simulink model "StereoImageRectificationHDL"  (R2022a)
settings: Solver=FixedStepDiscrete  StartTime=0.0  StopTime=totalPixels*totalLines  FixedStep=1  RelTol=1e-3
InitFcn:
  | load('stereoParams.mat');
  | img = imread(get_param('StereoImageRectificationHDL/LeftInputImage','FileName'));
  | dimOut=size(img);
  | [imgRowSize, imgColSize] = size(img);
  | run('ComputeRectificationParams.m');
values from neighbouring files (symbols this model uses):
  displacement = maxDev+firstRow    [ComputeRectificationParams.m]
  distCoeffsL = [this.CameraParameters1.RadialDistortion, this.CameraParameters1.TangentialDistortion]    [ComputeRectificationParams.m]
  distCoeffsR = [this.CameraParameters2.RadialDistortion, this.CameraParameters2.TangentialDistortion]    [ComputeRectificationParams.m]
  offset = displacement+50    [ComputeRectificationParams.m]
  recleftfx = 1/intrinsicL(1,1)    [ComputeRectificationParams.m]
  recleftfy = 1/intrinsicL(2,2)    [ComputeRectificationParams.m]
  recrightfx = 1/intrinsicR(1,1)    [ComputeRectificationParams.m]
  recrightfy = 1/intrinsicR(2,2)    [ComputeRectificationParams.m]
  totalLines = R + 100    (= 580)    [setup.m]
  totalPixels = C + frontPorch    (= 802)    [setup.m]
undefined symbols (not defined in the file or in its folder): gray, imgColSize, imgRowSize, intrinsicL, intrinsicR, leftH, rightH, XBounds, YBounds
libraries: simulink x62, hdlsllib x30, visionhdlio x4, visionsources x2, visionhdlutilities x1
(part 1 of 3)
settings Model: DataTypeOverride=Off  SimulationMode=accelerator  Creator=The MathWorks, Inc.  LastModifiedBy=kaputa
settings SolverCC: AlgebraicLoopSolver=TrustRegion
settings DataIOCC: SaveOutput=off  SaveTime=off
settings OptimizationCC: BlockReduction=off  ConditionallyExecuteInputs=off  DefaultParameterBehavior=Inlined
settings DebuggingCC: AlgebraicLoopMsg=error  SingleTaskRateTransMsg=error  ParameterPrecisionLossMsg=none  UnconnectedInputMsg=warning  UnconnectedOutputMsg=warning  UnconnectedLineMsg=warning  SFMachineParentedDataDiag=warning
settings HardwareCC: ProdBitPerPointer=32  ProdBitPerSizeT=32  ProdBitPerPtrDiffT=32  ProdLargestAtomicFloat=None  ProdIntDivRoundTo=Undefined  ProdEndianess=Unspecified  ProdWordSize=32  ProdHWDeviceType=ASIC/FPGA->ASIC/FPGA  TargetBitPerPointer=64  TargetBitPerSizeT=64  TargetBitPerPtrDiffT=64  TargetLongLongMode=on  TargetIntDivRoundTo=Zero  TargetEndianess=LittleEndian  TargetWordSize=64  TargetHWDeviceType=Custom Processor->MATLAB Host Computer  ProdEqTarget=off

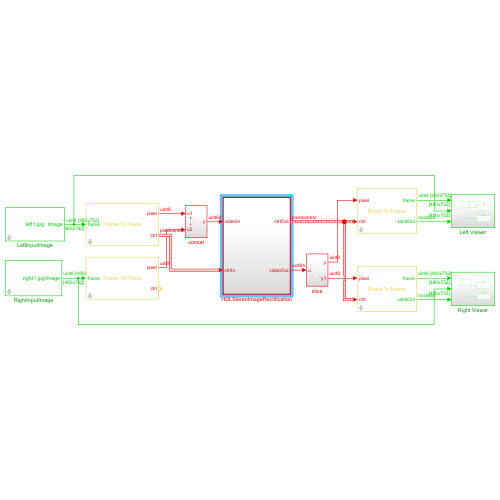
[thumbnail: Simulink's stored preview of the top-level diagram]
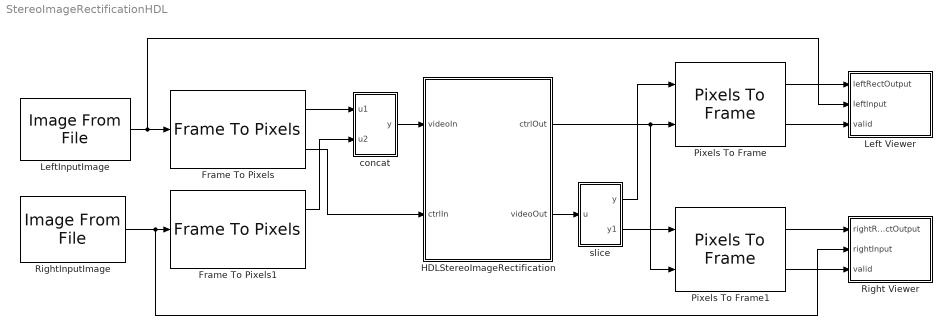
== system StereoImageRectificationHDL ==
  Frame To Pixels : visionhdlio/Frame To Pixels  NumComponents=1  NumPixels=1  VideoFormat=Custom  ActivePixelsPerLine=C  ActiveVideoLines=R  TotalPixelsPerLine=totalPixels  TotalVideoLines=totalLines  StartingActiveLine=topPorch  FrontPorch=frontPorch  SampleTime=0  VideoFormatCache=Custom  ActivePixelsPerLineCache=C  ActiveVideoLinesCache=R  TotalPixelsPerLineCache=totalPixels  TotalVideoLinesCache=totalLines  StartingActiveLineCache=topPorch  FrontPorchCache=frontPorch
      settings: SourceProductBaseCode=VT
  Frame To Pixels1 : visionhdlio/Frame To Pixels  NumComponents=1  NumPixels=1  VideoFormat=Custom  ActivePixelsPerLine=C  ActiveVideoLines=R  TotalPixelsPerLine=totalPixels  TotalVideoLines=totalLines  StartingActiveLine=topPorch  FrontPorch=frontPorch  SampleTime=0  VideoFormatCache=Custom  ActivePixelsPerLineCache=C  ActiveVideoLinesCache=R  TotalPixelsPerLineCache=totalPixels  TotalVideoLinesCache=totalLines  StartingActiveLineCache=topPorch  FrontPorchCache=frontPorch
      settings: SourceProductBaseCode=VT
  HDLStereoImageRectification : Subsystem  TreatAsAtomicUnit=on
  Left Viewer : Subsystem
  LeftInputImage : visionsources/Image From File  Tag=vipblks_nd  FileName=left1.jpg  Ts=totalPixels*totalLines  imagePorts=One multidimensional signal  OutPortLabels=R|G|B  ImageDataType=Inherit from input image  sdImageDataType=uint(8)  Signed=on  WordLength=16  FractionLengthMode=User-defined  FractionLength=15
  Pixels To Frame : visionhdlio/Pixels To Frame  NumComponents=1  NumPixels=1  VideoFormat=Custom  ActivePixelsPerLine=C  ActiveVideoLines=R  TotalPixelsPerLine=totalPixels  TotalVideoLines=totalLines  VideoFormatCache=Custom  ActivePixelsPerLineCache=C  ActiveVideoLinesCache=R  TotalPixelsPerLineCache=totalPixels  TotalVideoLinesCache=totalLines
      settings: SourceProductBaseCode=VT
  Pixels To Frame1 : visionhdlio/Pixels To Frame  NumComponents=1  NumPixels=1  VideoFormat=Custom  ActivePixelsPerLine=C  ActiveVideoLines=R  TotalPixelsPerLine=totalPixels  TotalVideoLines=totalLines  VideoFormatCache=Custom  ActivePixelsPerLineCache=C  ActiveVideoLinesCache=R  TotalPixelsPerLineCache=totalPixels  TotalVideoLinesCache=totalLines
      settings: SourceProductBaseCode=VT
  Right Viewer : Subsystem
  RightInputImage : visionsources/Image From File  Tag=vipblks_nd  FileName=right1.jpg  Ts=totalPixels*totalLines  imagePorts=One multidimensional signal  OutPortLabels=R|G|B  ImageDataType=Inherit from input image  sdImageDataType=uint(8)  Signed=on  WordLength=16  FractionLengthMode=User-defined  FractionLength=15
  concat : Subsystem
  slice : Subsystem
  wires:
  HDLStereoImageRectification/1(ctrlOut) -> Pixels To Frame1/2, Pixels To Frame/2
  Pixels To Frame/1 -> Left Viewer/1(leftRectOutput)
  Pixels To Frame/2 -> Left Viewer/3(valid)
  Pixels To Frame1/1 -> Right Viewer/1(rightRectOutput)
  Pixels To Frame1/2 -> Right Viewer/3(valid)
  LeftInputImage/1 -> Left Viewer/2(leftInput), Frame To Pixels/1
  RightInputImage/1 -> Right Viewer/2(rightInput), Frame To Pixels1/1
  Frame To Pixels/2 -> HDLStereoImageRectification/2(ctrlIn)
  Frame To Pixels/1 -> concat/1(u1)
  Frame To Pixels1/1 -> concat/2(u2)
  concat/1(y) -> HDLStereoImageRectification/1(videoIn)
  HDLStereoImageRectification/2(videoOut) -> slice/1(u)
  slice/1(y) -> Pixels To Frame/1
  slice/2(y1) -> Pixels To Frame1/1

== system StereoImageRectificationHDL/HDLStereoImageRectification ==
  videoIn : Inport
  ctrlIn : Inport  Port=2
  Bit Concat1 : hdlsllib/Logic and Bit Operations/Bit Concat  numInputs=4
  Bit Concat2 : hdlsllib/Logic and Bit Operations/Bit Concat  numInputs=4
  Bit Concat3 : hdlsllib/Logic and Bit Operations/Bit Concat  numInputs=2
  Compare To Constant : simulink/Logic and Bit Operations/Compare To Constant  relop===  const=40  OutDataTypeStr=boolean
  Constant : Constant  Value=0  OutDataTypeStr=Inherit: Inherit via back propagation  SampleTime=-1
  Delay8 : Delay  DelayLength=63
  GenerateControl : Subsystem
  LeftInterpolation : Subsystem
  LeftInverseGeometricTransform : Subsystem  mask{H=leftH}
      mask prompts: H "Inverse Homography Matrix"
  LeftUndistortion : Subsystem  mask{intrinsic=intrinsicL, distCoeffs=distCoeffsL, recfx=recleftfx, recfy=recleftfy}
      mask prompts: intrinsic "Camera intrinsic matrix"; distCoeffs "Distortion Coefficients"; recfx "Reciprocal of fx"; recfy "Reciprocal of fy"
  RectifiedCoordinateGeneration : Subsystem
  RightInterpolation : Subsystem
  RightInverseGeometricTransform : Subsystem  mask{H=rightH}
      mask prompts: H "Inverse Homography Matrix"
  RightUndistortion : Subsystem  mask{intrinsic=intrinsicR, distCoeffs=distCoeffsR, recfx=recrightfx, recfy=recrightfy}
      mask prompts: intrinsic "Camera intrinsic matrix"; distCoeffs "Distortion Coefficients"; recfx "Reciprocal of fx"; recfy "Reciprocal of fy"
  Switch : Switch  Criteria=u2 ~= 0  SaturateOnIntegerOverflow=off  InputSameDT=off
  Switch1 : Switch  Criteria=u2 ~= 0  SaturateOnIntegerOverflow=off  InputSameDT=off
  slice 1 : hdlsllib/Logic and Bit Operations/Bit Slice  lidx=31  ridx=24
      settings: SourceProductBaseCode=SL
  slice 2 : hdlsllib/Logic and Bit Operations/Bit Slice  lidx=63  ridx=56
      settings: SourceProductBaseCode=SL
  ctrlOut : Outport
  videoOut : Outport  Port=2
  wires:
  Bit Concat3/1 -> videoOut/1
  LeftInterpolation/2(leftCtrl) -> ctrlOut/1
  GenerateControl/1(ctrlOut) -> RectifiedCoordinateGeneration/1(ctrl)
  slice 1/1 -> LeftInterpolation/2(leftInputPixel)
  slice 2/1 -> RightInterpolation/2(rightInputPixel)
  videoIn/1 -> slice 2/1, slice 1/1
  ctrlIn/1 -> LeftInterpolation/1(leftInputCtrl), RightInterpolation/1(rightInputCtrl), GenerateControl/2(rightCtrlIn), GenerateControl/1(leftCtrlIn)
  LeftInverseGeometricTransform/1(x) -> LeftUndistortion/1(x)
  LeftInverseGeometricTransform/2(y) -> LeftUndistortion/2(y)
  LeftInverseGeometricTransform/3(ctrlOut) -> LeftUndistortion/3(ctrlIn)
  RightInverseGeometricTransform/1(x) -> RightUndistortion/1(x)
  RightInverseGeometricTransform/2(y) -> RightUndistortion/2(y)
  RightInverseGeometricTransform/3(ctrlOut) -> RightUndistortion/3(ctrlIn)
  RectifiedCoordinateGeneration/1(col) -> RightInverseGeometricTransform/1(col), LeftInverseGeometricTransform/1(col)
  RectifiedCoordinateGeneration/2(row) -> RightInverseGeometricTransform/2(row), Delay8/1, LeftInverseGeometricTransform/2(row)
  RectifiedCoordinateGeneration/3(ctrlOut) -> RightInverseGeometricTransform/3(ctrlIn), LeftInverseGeometricTransform/3(ctrlIn)
  LeftUndistortion/1(u) -> LeftInterpolation/3(u)
  LeftUndistortion/2(v) -> LeftInterpolation/4(v)
  LeftUndistortion/3("ctrlOut ") -> LeftInterpolation/5(ctrlIn)
  RightUndistortion/1(u) -> RightInterpolation/3(u)
  RightUndistortion/2(v) -> RightInterpolation/4(v)
  RightUndistortion/3("ctrlOut ") -> RightInterpolation/5(ctrlIn)
  Switch/1 -> Bit Concat1/1, Bit Concat1/2, Bit Concat1/3, Bit Concat1/4
  Delay8/1 -> Compare To Constant/1
  Compare To Constant/1 -> Switch/2, Switch1/2
  Constant/1 -> Switch1/1, Switch/1
  LeftInterpolation/1(leftPixel) -> Switch/3
  Switch1/1 -> Bit Concat2/4, Bit Concat2/3, Bit Concat2/2, Bit Concat2/1
  RightInterpolation/1(rightPixel) -> Switch1/3
  Bit Concat1/1 -> Bit Concat3/2
  Bit Concat2/1 -> Bit Concat3/1

== system StereoImageRectificationHDL/Left Viewer ==
  leftRectOutput : Inport
  leftInput : Inport  Port=2
  valid : Inport  Port=3
  Enabled Subsystem : Subsystem  TreatAsAtomicUnit=on
  Enabled Subsystem1 : Subsystem  TreatAsAtomicUnit=on
  wires:
  leftInput/1 -> Enabled Subsystem/1(In1)
  leftRectOutput/1 -> Enabled Subsystem1/1(In1)
  valid/1 -> Enabled Subsystem1/Enable, Enabled Subsystem/Enable

== system StereoImageRectificationHDL/Right Viewer ==
  rightRectOutput : Inport
  rightInput : Inport  Port=2
  valid : Inport  Port=3
  Enabled Subsystem : Subsystem  TreatAsAtomicUnit=on
  Enabled Subsystem1 : Subsystem  TreatAsAtomicUnit=on
  wires:
  valid/1 -> Enabled Subsystem/Enable, Enabled Subsystem1/Enable
  rightRectOutput/1 -> Enabled Subsystem1/1(In1)
  rightInput/1 -> Enabled Subsystem/1(In1)

== system StereoImageRectificationHDL/concat ==
  u1 : Inport
  u2 : Inport  Port=2
  Bit Concat1 : hdlsllib/Logic and Bit Operations/Bit Concat  numInputs=4
  Bit Concat2 : hdlsllib/Logic and Bit Operations/Bit Concat  numInputs=4
  Bit Concat3 : hdlsllib/Logic and Bit Operations/Bit Concat  numInputs=2
  y : Outport
  wires:
  u1/1 -> Bit Concat1/1, Bit Concat1/4, Bit Concat1/3, Bit Concat1/2
  Bit Concat2/1 -> Bit Concat3/1
  u2/1 -> Bit Concat2/1, Bit Concat2/2, Bit Concat2/3, Bit Concat2/4
  Bit Concat1/1 -> Bit Concat3/2
  Bit Concat3/1 -> y/1

== system StereoImageRectificationHDL/slice ==
  u : Inport
  slice 1 : hdlsllib/Logic and Bit Operations/Bit Slice  lidx=31  ridx=24
      settings: SourceProductBaseCode=SL
  slice 2 : hdlsllib/Logic and Bit Operations/Bit Slice  lidx=63  ridx=56
      settings: SourceProductBaseCode=SL
  y : Outport
  y1 : Outport  Port=2
  wires:
  slice 1/1 -> y/1
  u/1 -> slice 2/1, slice 1/1
  slice 2/1 -> y1/1

== system StereoImageRectificationHDL/HDLStereoImageRectification/GenerateControl ==
  note: modified to make the output control lines depend on the input valid signal.. at leat until the input image is all read in.
  leftCtrlIn : Inport
  rightCtrlIn : Inport  Port=2
  Bus Selector1 : BusSelector  OutputSignals=valid,vStart
  Compare To Constant : simulink/Logic and Bit Operations/Compare To Constant  relop=>  const=displacement  OutDataTypeStr=boolean
  Compare To Constant1 : simulink/Logic and Bit Operations/Compare To Constant  relop=>  const=(752*480)-(displacement*752)-2  OutDataTypeStr=boolean
  HDL Counter1 : hdlsllib/Sources/HDL Counter  CountType=Free running  CountInit=0  CountStep=1  CountMax=59  CountFromType=Initial value  CountFrom=0  CountResetPort=on  CountLoadPort=off  CountEnbPort=on  CountDirPort=off  CountHitOutputPort=off  CountDataType=Unsigned  CountWordLen=ceil(log2(dimOut(1)*dimOut(2)))  CountFracLen=0  CountSampTime=1
  Input : Subsystem
  Logical Operator : Logic  AllPortsSameDT=off  OutDataTypeStr=boolean
  Logical Operator1 : Logic  Operator=OR  AllPortsSameDT=off  OutDataTypeStr=boolean
  Logical Operator2 : Logic  Operator=OR  AllPortsSameDT=off  OutDataTypeStr=boolean
  PixelBusGenerator : Subsystem  mask{hEnd=dimOut(2)-1, vEnd=dimOut(1)*dimOut(2) - 1}
      mask prompts: hEnd "hEnd Count"; vEnd "vEnd Count"
      mask DialogControl DescGroupVar Prompt: Counter Values
  Scope : Scope  NumInputPorts=2
  ctrlOut : Outport
  wires:
  leftCtrlIn/1 -> Input/1(leftCtrlIn)
  rightCtrlIn/1 -> Bus Selector1/1, Input/2(rightCtrlIn)
  PixelBusGenerator/1(busOut) -> ctrlOut/1
  Input/1(rowCount) -> Compare To Constant/1
  Compare To Constant/1 -> Logical Operator/1
  Bus Selector1/1 -> Scope/1, Logical Operator/2  "<valid>"
  Logical Operator/1 -> Logical Operator1/1
  HDL Counter1/1 -> Compare To Constant1/1
  Compare To Constant1/1 -> Logical Operator1/2
  Logical Operator1/1 -> Scope/2, PixelBusGenerator/1(validIn), HDL Counter1/2
  Bus Selector1/2 -> Logical Operator2/2  "<vStart>"
  PixelBusGenerator/2(frameDone) -> Logical Operator2/1
  Logical Operator2/1 -> HDL Counter1/1

== system StereoImageRectificationHDL/HDLStereoImageRectification/LeftInterpolation ==
  leftInputCtrl : Inport
  leftInputPixel : Inport  Port=2
  u : Inport  Port=3
  v : Inport  Port=4
  ctrlIn : Inport  Port=5
  AddressGeneration : Subsystem
  BilinearInterpolation : Subsystem
  CacheMemory : Subsystem
  leftPixel : Outport
  leftCtrl : Outport  Port=2
  wires:
  BilinearInterpolation/2(rectCtrl) -> leftCtrl/1
  u/1 -> AddressGeneration/1(u)
  AddressGeneration/3(index) -> BilinearInterpolation/3(Index)
  AddressGeneration/2(leftAdd) -> [leftAdd]
  AddressGeneration/1(deltaU) -> BilinearInterpolation/1(deltaU)
  AddressGeneration/4(deltaV) -> BilinearInterpolation/4(deltaV)
  ctrlIn/1 -> AddressGeneration/3(ctrl)
  AddressGeneration/5(ctrlOut) -> BilinearInterpolation/5(ctrlIn)
  [leftPixel] -> BilinearInterpolation/2(pixValue)
  v/1 -> AddressGeneration/2(v)
  leftInputPixel/1 -> CacheMemory/1(pixel)
  leftInputCtrl/1 -> CacheMemory/2(ctrl)
  CacheMemory/1(pixValue) -> [leftPixel]
  [leftAdd] -> CacheMemory/3(readAddr)
  BilinearInterpolation/1(rectPixel) -> leftPixel/1

== system StereoImageRectificationHDL/HDLStereoImageRectification/LeftInverseGeometricTransform ==
  col : Inport
  row : Inport  Port=2
  ctrlIn : Inport  Port=3
  Data Type Conversion : DataTypeConversion  OutDataTypeStr=fixdt(1,ceil(log2(max(dimOut(1),dimOut(2))))+2+24,24)  RndMeth=Nearest  SaturateOnIntegerOverflow=off
  Data Type Conversion1 : DataTypeConversion  OutDataTypeStr=fixdt(1,ceil(log2(max(dimOut(1),dimOut(2))))+2+24,24)  RndMeth=Nearest  SaturateOnIntegerOverflow=off
  Delay29 : Delay  DelayLength=9+1+2
  Transformation : Subsystem
  x : Outport
  y : Outport  Port=2
  ctrlOut : Outport  Port=3
  wires:
  ctrlIn/1 -> Delay29/1
  col/1 -> Transformation/1(col)
  row/1 -> Transformation/2(row)
  Transformation/1(x) -> Data Type Conversion/1
  Transformation/2(y) -> Data Type Conversion1/1
  Delay29/1 -> ctrlOut/1
  Data Type Conversion/1 -> x/1
  Data Type Conversion1/1 -> y/1

== system StereoImageRectificationHDL/HDLStereoImageRectification/LeftUndistortion ==
  x : Inport
  y : Inport  Port=2
  ctrlIn : Inport  Port=3
  Delay32 : Delay  DelayLength=22
  Denormalization : Subsystem
  Normalization : Subsystem
  ParameterCalculation : Subsystem
  RadialDistortion : Subsystem
  dxTangential : Subsystem
  dyTangential : Subsystem
  u : Outport
  v : Outport  Port=2
  "ctrlOut " : Outport  Port=3
  wires:
  Normalization/2(xNorm) -> ParameterCalculation/2(xNorm), Denormalization/5(xNorm)
  ParameterCalculation/3(xyProduct) -> dyTangential/2(xyProd), dxTangential/2(xyProd)
  ParameterCalculation/4(xNorm2) -> dxTangential/3(xNorm2)
  ParameterCalculation/5(yNorm2) -> dyTangential/3(yNorm2)
  Normalization/1(yNorm) -> Denormalization/1(yNorm), ParameterCalculation/1(yNorm)
  ctrlIn/1 -> Delay32/1
  Delay32/1 -> "ctrlOut "/1
  y/1 -> Normalization/1(yCoordinate)
  x/1 -> Normalization/2(xCoordinate)
  Denormalization/1(v) -> v/1
  Denormalization/2(u) -> u/1
  RadialDistortion/1(alpha) -> Denormalization/2(alpha)
  dxTangential/1(dxTan) -> Denormalization/3(dxTan)
  dyTangential/1(dyTan) -> Denormalization/4(dyTan)
  ParameterCalculation/2(r2) -> dyTangential/1(r2), dxTangential/1(r2), RadialDistortion/2(r2)
  ParameterCalculation/1(r4) -> RadialDistortion/1(r4)

== system StereoImageRectificationHDL/HDLStereoImageRectification/RectifiedCoordinateGeneration ==
  ctrl : Inport
  Compare To Constant1 : simulink/Logic and Bit Operations/Compare To Constant  relop===  const=YBounds(2)+1  OutDataTypeStr=boolean
  Compare To Constant2 : simulink/Logic and Bit Operations/Compare To Constant  relop===  const=XBounds(2)  OutDataTypeStr=boolean
  Compare To Constant3 : simulink/Logic and Bit Operations/Compare To Constant  relop=>=  const=YBounds(2)+1  OutDataTypeStr=boolean
  Delay16 : Delay  DelayLength=1
  HDL Counter3 : hdlsllib/Sources/HDL Counter  CountType=Count limited  CountInit=XBounds(1)  CountStep=1  CountMax=XBounds(2)  CountFromType=Initial value  CountFrom=XBounds(1)  CountResetPort=on  CountLoadPort=off  CountEnbPort=on  CountDirPort=off  CountHitOutputPort=off  CountDataType=Signed  CountWordLen=ceil(log2(max(abs(XBounds(1)), abs(XBounds(2)))))+1  CountFracLen=0  CountSampTime=1
  HDL Counter4 : hdlsllib/Sources/HDL Counter  CountType=Count limited  CountInit=YBounds(1)  CountStep=1  CountMax=YBounds(2)+2  CountFromType=Initial value  CountFrom=YBounds(1)  CountResetPort=on  CountLoadPort=off  CountEnbPort=on  CountDirPort=off  CountHitOutputPort=off  CountDataType=Signed  CountWordLen=ceil(log2(max(abs(YBounds(1)), abs(YBounds(2)+2))))+1  CountFracLen=0  CountSampTime=1
  Logical Operator2 : Logic  AllPortsSameDT=off  OutDataTypeStr=boolean
  Pixel Control Bus Selector : BusSelector  OutputSignals=valid
  col : Outport
  row : Outport  Port=2
  ctrlOut : Outport  Port=3
  wires:
  Delay16/1 -> HDL Counter4/1
  Compare To Constant2/1 -> Logical Operator2/2
  Pixel Control Bus Selector/1 -> Logical Operator2/1, HDL Counter3/2  "<valid>"
  ctrl/1 -> ctrlOut/1, Pixel Control Bus Selector/1
  Compare To Constant1/1 -> Delay16/1
  HDL Counter3/1 -> Compare To Constant2/1, col/1  "C"
  Compare To Constant3/1 -> HDL Counter3/1
  HDL Counter4/1 -> Compare To Constant3/1, Compare To Constant1/1, row/1  "R"
  Logical Operator2/1 -> HDL Counter4/2

== system StereoImageRectificationHDL/HDLStereoImageRectification/RightInterpolation ==
  rightInputCtrl : Inport
  rightInputPixel : Inport  Port=2
  u : Inport  Port=3
  v : Inport  Port=4
  ctrlIn : Inport  Port=5
  AddressGeneration : Subsystem
  BilinearInterpolation : Subsystem
  CacheMemory : Subsystem
  rightPixel : Outport
  rightCtrl : Outport  Port=2
  wires:
  AddressGeneration/5(ctrlOut) -> BilinearInterpolation/5(ctrlIn)
  v/1 -> AddressGeneration/2(v)
  AddressGeneration/2(leftAdd) -> [rightAdd]
  [rightPixel] -> BilinearInterpolation/2(pixValue)
  AddressGeneration/1(deltaU) -> BilinearInterpolation/1(deltaU)
  ctrlIn/1 -> AddressGeneration/3(ctrl)
  AddressGeneration/3(index) -> BilinearInterpolation/3(Index)
  BilinearInterpolation/2(rightctrl) -> rightCtrl/1
  AddressGeneration/4(deltaV) -> BilinearInterpolation/4(deltaV)
  u/1 -> AddressGeneration/1(u)
  BilinearInterpolation/1(rightPixel) -> rightPixel/1
  rightInputPixel/1 -> CacheMemory/1(rightPixel1)
  rightInputCtrl/1 -> CacheMemory/2(rightCtrl1)
  CacheMemory/1(rightPixValue) -> [rightPixel]
  [rightAdd] -> CacheMemory/3(rightReadAddr)

== system StereoImageRectificationHDL/HDLStereoImageRectification/RightInverseGeometricTransform ==
  col : Inport
  row : Inport  Port=2
  ctrlIn : Inport  Port=3
  Data Type Conversion : DataTypeConversion  OutDataTypeStr=fixdt(1,ceil(log2(max(dimOut(1),dimOut(2))))+2+24,24)  RndMeth=Nearest  SaturateOnIntegerOverflow=off
  Data Type Conversion1 : DataTypeConversion  OutDataTypeStr=fixdt(1,ceil(log2(max(dimOut(1),dimOut(2))))+2+24,24)  RndMeth=Nearest  SaturateOnIntegerOverflow=off
  Delay29 : Delay  DelayLength=9+1+2
  Transformation : Subsystem
  x : Outport
  y : Outport  Port=2
  ctrlOut : Outport  Port=3
  wires:
  ctrlIn/1 -> Delay29/1
  col/1 -> Transformation/1(col)
  row/1 -> Transformation/2(row)
  Transformation/1(x) -> Data Type Conversion/1
  Transformation/2(y) -> Data Type Conversion1/1
  Delay29/1 -> ctrlOut/1
  Data Type Conversion/1 -> x/1
  Data Type Conversion1/1 -> y/1

== system StereoImageRectificationHDL/HDLStereoImageRectification/RightUndistortion ==
  x : Inport
  y : Inport  Port=2
  ctrlIn : Inport  Port=3
  Delay32 : Delay  DelayLength=22
  Denormalization : Subsystem
  Normalization : Subsystem
  ParameterCalculation : Subsystem
  RadialDistortion : Subsystem
  dxTangential : Subsystem
  dyTangential : Subsystem
  u : Outport
  v : Outport  Port=2
  "ctrlOut " : Outport  Port=3
  wires:
  ParameterCalculation/1(r4) -> RadialDistortion/1(r4)
  ParameterCalculation/2(r2) -> RadialDistortion/2(r2), dxTangential/1(r2), dyTangential/1(r2)
  dyTangential/1(dyTan) -> Denormalization/4(dyTan)
  dxTangential/1(dxTan) -> Denormalization/3(dxTan)
  RadialDistortion/1(alpha) -> Denormalization/2(alpha)
  Denormalization/2(u) -> u/1
  Denormalization/1(v) -> v/1
  x/1 -> Normalization/2(xCoordinate)
  y/1 -> Normalization/1(yCoordinate)
  Delay32/1 -> "ctrlOut "/1
  ctrlIn/1 -> Delay32/1
  Normalization/1(yNorm) -> ParameterCalculation/1(yNorm), Denormalization/1(yNorm)
  ParameterCalculation/5(yNorm2) -> dyTangential/3(yNorm2)
  ParameterCalculation/4(xNorm2) -> dxTangential/3(xNorm2)
  ParameterCalculation/3(xyProduct) -> dxTangential/2(xyProd), dyTangential/2(xyProd)
  Normalization/2(xNorm) -> Denormalization/5(xNorm), ParameterCalculation/2(xNorm)

== system StereoImageRectificationHDL/Left Viewer/Enabled Subsystem ==
  In1 : Inport
  Enable : EnablePort
  LeftInputImage : VideoViewer  colormapValue=gray(256)  FigPos=[1 718 1280 622.666666666667]
  wires:
  In1/1 -> LeftInputImage/1

== system StereoImageRectificationHDL/Left Viewer/Enabled Subsystem1 ==
  In1 : Inport
  Enable : EnablePort
  LeftRectifiedImage : VideoViewer  colormapValue=gray(256)  FigPos=[-2655 959.333333333333 1280 622.666666666667]
  wires:
  In1/1 -> LeftRectifiedImage/1

== system StereoImageRectificationHDL/Right Viewer/Enabled Subsystem ==
  In1 : Inport
  Enable : EnablePort
  RightInputImage : VideoViewer  colormapValue=gray(256)  FigPos=[-43.6666666666667 820 1280 622.666666666667]
  wires:
  In1/1 -> RightInputImage/1

== system StereoImageRectificationHDL/Right Viewer/Enabled Subsystem1 ==
  In1 : Inport
  Enable : EnablePort
  RightRectifiedImage : VideoViewer  colormapValue=gray(256)  FigPos=[25 706 1097.33333333333 520]
  wires:
  In1/1 -> RightRectifiedImage/1

== system StereoImageRectificationHDL/HDLStereoImageRectification/GenerateControl/Input ==
  leftCtrlIn : Inport
  rightCtrlIn : Inport  Port=2
  Bus Selector : BusSelector  OutputSignals=hStart,valid,vEnd
  Bus Selector1 : BusSelector  OutputSignals=hStart,vEnd,valid
  Constant : Constant  Value=0  OutDataTypeStr=boolean  SampleTime=-1
  HDL Counter1 : hdlsllib/Sources/HDL Counter  CountType=Free running  CountInit=0  CountStep=1  CountMax=(imgColSize*imgRowSize) - 1  CountFromType=Initial value  CountFrom=0  CountResetPort=on  CountLoadPort=off  CountEnbPort=on  CountDirPort=off  CountHitOutputPort=off  CountDataType=Unsigned  CountWordLen=ceil(log2(imgRowSize+1))  CountFracLen=0  CountSampTime=1
  Logical Operator : Logic  AllPortsSameDT=off  OutDataTypeStr=boolean
  Logical Operator1 : Logic  AllPortsSameDT=off  OutDataTypeStr=boolean
  Logical Operator4 : Logic  AllPortsSameDT=off  OutDataTypeStr=boolean
  Switch : Switch  Criteria=u2 ~= 0  SaturateOnIntegerOverflow=off  InputSameDT=off
  rowCount : Outport  VectorParamsAs1DForOutWhenUnconnected=off
  wires:
  Bus Selector1/1 -> Logical Operator/2  "<hStart>"
  leftCtrlIn/1 -> Bus Selector/1
  rightCtrlIn/1 -> Bus Selector1/1
  Logical Operator4/1 -> Switch/2
  Logical Operator/1 -> Switch/1
  Constant/1 -> Switch/3
  Bus Selector1/3 -> Logical Operator4/2  "<valid>"
  Bus Selector/2 -> Logical Operator4/1  "<valid>"
  Logical Operator1/1 -> HDL Counter1/1  "<vEnd>"
  Switch/1 -> HDL Counter1/2
  HDL Counter1/1 -> rowCount/1
  Bus Selector/1 -> Logical Operator/1  "<hStart>"
  Bus Selector1/2 -> Logical Operator1/2  "<vEnd>"
  Bus Selector/3 -> Logical Operator1/1  "<vEnd>"

== system StereoImageRectificationHDL/HDLStereoImageRectification/GenerateControl/PixelBusGenerator ==
  validIn : Inport
  Horizontal : hdlsllib/Sources/HDL Counter  CountType=Count limited  CountInit=0  CountStep=1  CountMax=hEnd  CountFromType=Initial value  CountFrom=0  CountResetPort=off  CountLoadPort=off  CountEnbPort=on  CountDirPort=off  CountHitOutputPort=off  CountDataType=Unsigned  CountWordLen=ceil(log2(hEnd))  CountFracLen=0  CountSampTime=1
  Logical Operator{3..6} (4 alike) : Logic  AllPortsSameDT=off  OutDataTypeStr=boolean
  Pixel Control Bus Creator : visionhdlutilities/Pixel Control Bus Creator
      settings: SourceProductBaseCode=VT
  Vertical : hdlsllib/Sources/HDL Counter  CountType=Count limited  CountInit=0  CountStep=1  CountMax=vEnd  CountFromType=Initial value  CountFrom=0  CountResetPort=off  CountLoadPort=off  CountEnbPort=on  CountDirPort=off  CountHitOutputPort=off  CountDataType=Unsigned  CountWordLen=ceil(log2(vEnd))  CountFracLen=0  CountSampTime=1
  hEnd : simulink/Logic and Bit Operations/Compare To Constant  relop===  const=hEnd  OutDataTypeStr=boolean
  hStart : simulink/Logic and Bit Operations/Compare To Constant  relop===  const=0  OutDataTypeStr=boolean
  vEnd : simulink/Logic and Bit Operations/Compare To Constant  relop===  const=vEnd  OutDataTypeStr=boolean
  vStart : simulink/Logic and Bit Operations/Compare To Constant  relop===  const=0  OutDataTypeStr=boolean
  busOut : Outport  VectorParamsAs1DForOutWhenUnconnected=off
  frameDone : Outport  Port=2  VectorParamsAs1DForOutWhenUnconnected=off
  wires:
  validIn/1 -> Logical Operator4/1, Logical Operator5/1, Logical Operator6/1, Logical Operator3/1, Horizontal/1, Pixel Control Bus Creator/5, Vertical/1
  Horizontal/1 -> hStart/1, hEnd/1
  hEnd/1 -> Logical Operator4/2
  Vertical/1 -> vStart/1, vEnd/1
  vStart/1 -> Logical Operator5/2
  vEnd/1 -> Logical Operator6/2
  Logical Operator5/1 -> Pixel Control Bus Creator/3
  Logical Operator3/1 -> Pixel Control Bus Creator/1
  Logical Operator4/1 -> Pixel Control Bus Creator/2
  hStart/1 -> Logical Operator3/2
  Logical Operator6/1 -> Pixel Control Bus Creator/4, frameDone/1
  Pixel Control Bus Creator/1 -> busOut/1

== system StereoImageRectificationHDL/HDLStereoImageRectification/LeftInterpolation/AddressGeneration ==
  u : Inport
  v : Inport  Port=2
  ctrl : Inport  Port=3
  Add : Sum  Inputs=+-  OutDataTypeStr=Inherit: Inherit via back propagation
  Add1 : Sum  Inputs=+-  OutDataTypeStr=Inherit: Inherit via back propagation
  AddressCalculation : Subsystem
  Data Type Conversion : DataTypeConversion  OutDataTypeStr=fixdt(0,max(ceil(log2(max(dimOut))),16),0)  SaturateOnIntegerOverflow=off  RndMeth=Floor
  Data Type Conversion1 : DataTypeConversion  OutDataTypeStr=fixdt(0,max(ceil(log2(max(dimOut))),16),0)  SaturateOnIntegerOverflow=off  RndMeth=Floor
  Delay{,1..3,7} (5 alike) : Delay  DelayLength=1
  Delay4 : Delay  DelayLength=4+1+3+3+10
  Delay5 : Delay  DelayLength=4+3+3+10
  Delay6 : Delay  DelayLength=4+3+3+10
  deltaU : Outport
  leftAdd : Outport  Port=2
  index : Outport  Port=3
  deltaV : Outport  Port=4
  ctrlOut : Outport  Port=5
  wires:
  v/1 -> Delay2/1, Data Type Conversion1/1
  Data Type Conversion1/1 -> Delay3/1, AddressCalculation/2(row)
  Data Type Conversion/1 -> Delay1/1, AddressCalculation/1(col)
  u/1 -> Delay/1, Data Type Conversion/1
  Delay/1 -> Add/1
  Delay1/1 -> Add/2
  Add/1 -> Delay6/1  "deltaU"
  Delay3/1 -> Add1/2
  Add1/1 -> Delay5/1  "deltaV"
  Delay2/1 -> Add1/1
  AddressCalculation/1(leftAdd) -> leftAdd/1
  AddressCalculation/2(leftIndex) -> Delay7/1
  ctrl/1 -> Delay4/1
  Delay6/1 -> deltaU/1
  Delay7/1 -> index/1
  Delay5/1 -> deltaV/1
  Delay4/1 -> ctrlOut/1

== system StereoImageRectificationHDL/HDLStereoImageRectification/LeftInterpolation/BilinearInterpolation ==
  deltaU : Inport
  pixValue : Inport  Port=2
  Index : Inport  Port=3
  deltaV : Inport  Port=4
  ctrlIn : Inport  Port=5
  BilinearInterpolationEquation : Subsystem
  Constant : Constant  Value=0  OutDataTypeStr=Inherit: Inherit via back propagation  SampleTime=-1
  Delay8 : Delay  DelayLength=8
  IndexChangeForInterpolation : MATLAB Function  TreatAsAtomicUnit=on
  Pixel Control Bus Selector : BusSelector  OutputSignals=valid
  Switch : Switch  Criteria=u2 ~= 0  SaturateOnIntegerOverflow=off  InputSameDT=off
  rectPixel : Outport
  rectCtrl : Outport  Port=2
  wires:
  Switch/1 -> rectPixel/1
  IndexChangeForInterpolation/1(pixOut) -> BilinearInterpolationEquation/2(pixValue)
  Constant/1 -> Switch/3
  pixValue/1 -> IndexChangeForInterpolation/1(pixelValue)
  BilinearInterpolationEquation/1(leftPixel) -> Switch/1
  Pixel Control Bus Selector/1 -> Switch/2  "<valid>"
  Delay8/1 -> rectCtrl/1, Pixel Control Bus Selector/1
  deltaU/1 -> BilinearInterpolationEquation/1(deltaU)
  deltaV/1 -> BilinearInterpolationEquation/3(deltaV)
  Index/1 -> IndexChangeForInterpolation/2(index)
  ctrlIn/1 -> Delay8/1

== system StereoImageRectificationHDL/HDLStereoImageRectification/LeftInterpolation/CacheMemory ==
  pixel : Inport
  ctrl : Inport  Port=2
  readAddr : Inport  Port=3
  Data Type Conversion : DataTypeConversion  OutDataTypeStr=fixdt(0,ceil(log2(offset*dimOut(2)/4)),0)  SaturateOnIntegerOverflow=off  RndMeth=Floor
  Simple Dual Port RAM System : hdlsllib/HDL RAMs/Simple Dual Port RAM System  RAMType=Simple dual port  WriteOutputValue=New data  RAMInitialValue=0  SimulateUsing=Code generation
      settings: SourceProductBaseCode=SL
  WriteControl : Subsystem
  pixValue : Outport  VectorParamsAs1DForOutWhenUnconnected=off
  wires:
  readAddr/1 -> Data Type Conversion/1
  WriteControl/2(wr_addr) -> Simple Dual Port RAM System/2
  Simple Dual Port RAM System/1 -> pixValue/1
  ctrl/1 -> WriteControl/2(ctrl)
  WriteControl/1(din) -> Simple Dual Port RAM System/1
  Data Type Conversion/1 -> Simple Dual Port RAM System/4
  WriteControl/3(wr_en) -> Simple Dual Port RAM System/3
  pixel/1 -> WriteControl/1(pixel)

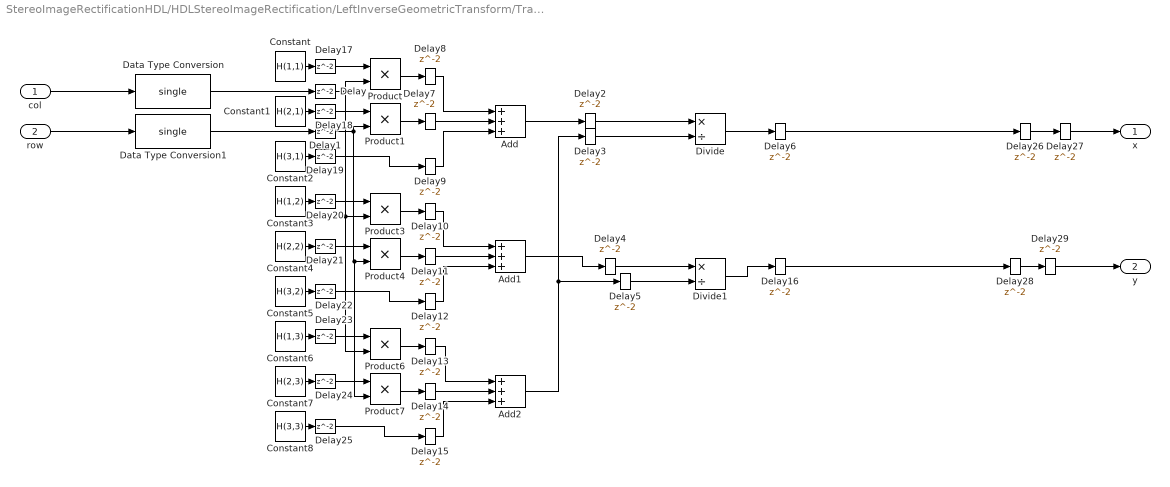
== system StereoImageRectificationHDL/HDLStereoImageRectification/LeftInverseGeometricTransform/Transformation ==
  col : Inport
  row : Inport  Port=2
  Add : Sum  Inputs=3  RndMeth=Round
  Add1 : Sum  Inputs=3  RndMeth=Round
  Add2 : Sum  Inputs=3  RndMeth=Round
  Constant : Constant  Value=H(1,1)  OutDataTypeStr=single  SampleTime=-1
  Constant1 : Constant  Value=H(2,1)  OutDataTypeStr=single  SampleTime=-1
  Constant2 : Constant  Value=H(3,1)  OutDataTypeStr=single  SampleTime=-1
  Constant3 : Constant  Value=H(1,2)  OutDataTypeStr=single  SampleTime=-1
  Constant4 : Constant  Value=H(2,2)  OutDataTypeStr=single  SampleTime=-1
  Constant5 : Constant  Value=H(3,2)  OutDataTypeStr=single  SampleTime=-1
  Constant6 : Constant  Value=H(1,3)  OutDataTypeStr=single  SampleTime=-1
  Constant7 : Constant  Value=H(2,3)  OutDataTypeStr=single  SampleTime=-1
  Constant8 : Constant  Value=H(3,3)  OutDataTypeStr=single  SampleTime=-1
  Data Type Conversion : DataTypeConversion  OutDataTypeStr=single  SaturateOnIntegerOverflow=off  RndMeth=Floor
  Data Type Conversion1 : DataTypeConversion  OutDataTypeStr=single  SaturateOnIntegerOverflow=off  RndMeth=Floor
  Delay{,1..29} (30 alike) : Delay
  Divide : Product  Inputs=*/
  Divide1 : Product  Inputs=*/
  Product{,1,3..4,6..7} (6 alike) : Product  RndMeth=Round
  x : Outport
  y : Outport  Port=2
  wires:
  Constant5/1 -> Delay22/1
  Product/1 -> Delay8/1
  Delay12/1 -> Add1/3
  Constant1/1 -> Delay18/1
  Constant6/1 -> Delay23/1
  Add2/1 -> Delay3/1, Delay5/1
  Constant3/1 -> Delay20/1
  Delay13/1 -> Add2/1
  Constant4/1 -> Delay21/1
  Delay21/1 -> Product4/1
  Add/1 -> Delay2/1
  Delay10/1 -> Add1/1
  Delay9/1 -> Add/3
  Delay25/1 -> Delay15/1
  Delay1/1 -> Product7/2, Product4/2, Product1/2
  Delay7/1 -> Add/2
  Delay14/1 -> Add2/2
  Delay/1 -> Product/2, Product6/2, Product3/2
  Delay15/1 -> Add2/3
  Product6/1 -> Delay13/1
  Constant7/1 -> Delay24/1
  Delay11/1 -> Add1/2
  Delay22/1 -> Delay12/1
  Constant2/1 -> Delay19/1
  Product4/1 -> Delay11/1
  Constant/1 -> Delay17/1
  Product1/1 -> Delay7/1
  Delay17/1 -> Product/1
  Product3/1 -> Delay10/1
  Product7/1 -> Delay14/1
  Delay20/1 -> Product3/1
  Delay24/1 -> Product7/1
  Delay18/1 -> Product1/1
  col/1 -> Data Type Conversion/1
  Delay19/1 -> Delay9/1
  Delay8/1 -> Add/1
  Constant8/1 -> Delay25/1
  Delay23/1 -> Product6/1
  row/1 -> Data Type Conversion1/1
  Data Type Conversion/1 -> Delay/1
  Data Type Conversion1/1 -> Delay1/1
  Delay6/1 -> Delay26/1
  Delay16/1 -> Delay28/1
  Divide/1 -> Delay6/1
  Divide1/1 -> Delay16/1
  Add1/1 -> Delay4/1
  Delay2/1 -> Divide/1
  Delay3/1 -> Divide/2
  Delay4/1 -> Divide1/1
  Delay5/1 -> Divide1/2
  Delay26/1 -> Delay27/1
  Delay27/1 -> x/1
  Delay28/1 -> Delay29/1
  Delay29/1 -> y/1

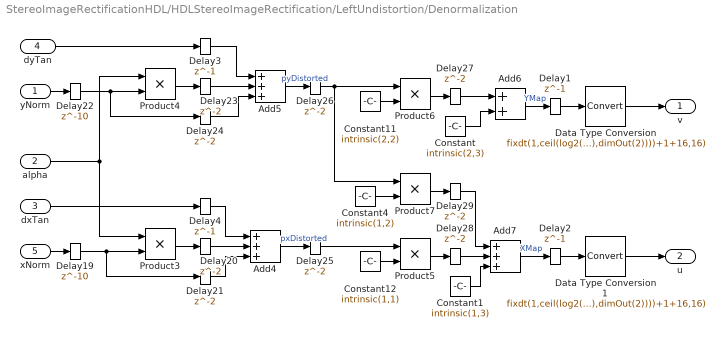
== system StereoImageRectificationHDL/HDLStereoImageRectification/LeftUndistortion/Denormalization ==
  yNorm : Inport
  alpha : Inport  Port=2
  dxTan : Inport  Port=3
  dyTan : Inport  Port=4
  xNorm : Inport  Port=5
  Add4 : Sum  Inputs=+++
  Add5 : Sum  Inputs=+++
  Add6 : Sum
  Add7 : Sum  Inputs=+++
  Constant : Constant  Value=intrinsic(2,3)  OutDataTypeStr=fixdt(1,ceil(log2(intrinsic(2,3)))+24,23)  SampleTime=-1
  Constant1 : Constant  Value=intrinsic(1,3)  OutDataTypeStr=fixdt(1,ceil(log2(intrinsic(1,3)))+24,23)  SampleTime=-1
  Constant11 : Constant  Value=intrinsic(2,2)  OutDataTypeStr=fixdt(1,ceil(log2(intrinsic(2,2)))+24,23)  SampleTime=-1
  Constant12 : Constant  Value=intrinsic(1,1)  OutDataTypeStr=fixdt(1,ceil(log2(intrinsic(1,1)))+24,23)  SampleTime=-1
  Constant4 : Constant  Value=intrinsic(1,2)  OutDataTypeStr=fixdt(1,17,16)  SampleTime=-1
  Data Type Conversion : DataTypeConversion  OutDataTypeStr=fixdt(1,ceil(log2(max(dimOut(1),dimOut(2))))+1+16,16)  RndMeth=Nearest  SaturateOnIntegerOverflow=off
  Data Type Conversion1 : DataTypeConversion  OutDataTypeStr=fixdt(1,ceil(log2(max(dimOut(1),dimOut(2))))+1+16,16)  RndMeth=Nearest  SaturateOnIntegerOverflow=off
  Delay{1..4} (4 alike) : Delay  DelayLength=1
  Delay19 : Delay  DelayLength=10
  Delay{20..21,23..29} (9 alike) : Delay
  Delay22 : Delay  DelayLength=10
  Product{3..7} (5 alike) : Product  OutDataTypeStr=Inherit: Same as first input
  v : Outport
  u : Outport  Port=2
  wires:
  xNorm/1 -> Delay19/1
  Delay25/1 -> Product5/1
  Delay20/1 -> Add4/2
  Product7/1 -> Delay29/1
  Delay22/1 -> Delay24/1, Product4/2
  alpha/1 -> Product4/1, Product3/1
  Constant4/1 -> Product7/2
  Add6/1 -> Delay1/1  "YMap"
  Delay21/1 -> Add4/3
  Constant1/1 -> Add7/3
  dyTan/1 -> Delay3/1
  Delay24/1 -> Add5/3
  Constant/1 -> Add6/2
  Product4/1 -> Delay23/1
  Product5/1 -> Delay28/1
  Add4/1 -> Delay25/1  "pxDistorted"
  Product6/1 -> Delay27/1
  Delay27/1 -> Add6/1
  Product3/1 -> Delay20/1
  Delay28/1 -> Add7/2
  Delay29/1 -> Add7/1
  Add5/1 -> Delay26/1  "pyDistorted"
  Add7/1 -> Delay2/1  "XMap"
  Constant11/1 -> Product6/2
  Delay26/1 -> Product7/1, Product6/1
  Constant12/1 -> Product5/2
  Delay19/1 -> Product3/2, Delay21/1
  Delay23/1 -> Add5/2
  yNorm/1 -> Delay22/1
  dxTan/1 -> Delay4/1
  Data Type Conversion/1 -> v/1
  Data Type Conversion1/1 -> u/1
  Delay3/1 -> Add5/1
  Delay4/1 -> Add4/1
  Delay1/1 -> Data Type Conversion/1
  Delay2/1 -> Data Type Conversion1/1

== system StereoImageRectificationHDL/HDLStereoImageRectification/LeftUndistortion/Normalization ==
  yCoordinate : Inport
  xCoordinate : Inport  Port=2
  Add : Sum  Inputs=+-
  Add1 : Sum  Inputs=+-
  Constant : Constant  Value=intrinsic(2,3)  OutDataTypeStr=fixdt(1,ceil(log2(intrinsic(2,3)))+24,23)  SampleTime=-1
  Constant1 : Constant  Value=intrinsic(1,3)  OutDataTypeStr=fixdt(1,ceil(log2(intrinsic(1,3)))+24,23)  SampleTime=-1
  Constant2 : Constant  Value=recfy  OutDataTypeStr=Inherit: Inherit via back propagation  SampleTime=-1
  Constant3 : Constant  Value=recfx  OutDataTypeStr=Inherit: Inherit via back propagation  SampleTime=-1
  Delay{1..3,8} (4 alike) : Delay
  Delay30 : Delay  DelayLength=1
  Delay31 : Delay  DelayLength=1
  Product13 : Product  OutDataTypeStr=Inherit: Same as first input
  Product14 : Product  OutDataTypeStr=Inherit: Same as first input
  yNorm : Outport
  xNorm : Outport  Port=2
  wires:
  Constant1/1 -> Add1/2
  Delay3/1 -> Product14/1
  Add1/1 -> Delay3/1
  Constant/1 -> Add/2
  Constant3/1 -> Product14/2
  Constant2/1 -> Product13/2
  yCoordinate/1 -> Delay30/1
  Delay8/1 -> Product13/1
  Delay31/1 -> Add1/1
  Delay30/1 -> Add/1
  Product13/1 -> Delay1/1  "yNorm"
  Add/1 -> Delay8/1
  Product14/1 -> Delay2/1  "xNorm"
  xCoordinate/1 -> Delay31/1
  Delay1/1 -> yNorm/1
  Delay2/1 -> xNorm/1

== system StereoImageRectificationHDL/HDLStereoImageRectification/LeftUndistortion/ParameterCalculation ==
  yNorm : Inport
  xNorm : Inport  Port=2
  Add2 : Sum
  Delay{1..4,6..7,9} (7 alike) : Delay
  Product{,10..12} (4 alike) : Product  OutDataTypeStr=Inherit: Inherit via back propagation
  r4 : Outport
  r2 : Outport  Port=2
  xyProduct : Outport  Port=3
  xNorm2 : Outport  Port=4
  yNorm2 : Outport  Port=5
  wires:
  Product10/1 -> Delay6/1  "yNorm2"
  Product11/1 -> Delay7/1  "xNorm2"
  Product12/1 -> r4/1  "r4"
  Delay9/1 -> Product12/1, r2/1, Product12/2
  Delay7/1 -> Delay4/1, Add2/2
  Delay6/1 -> Add2/1, Delay3/1
  Add2/1 -> Delay9/1  "r2"
  yNorm/1 -> Product10/1, Product10/2, Product/1
  Product/1 -> Delay1/1  "xyProduct"
  xNorm/1 -> Product11/2, Product11/1, Product/2
  Delay1/1 -> Delay2/1
  Delay2/1 -> xyProduct/1
  Delay3/1 -> yNorm2/1
  Delay4/1 -> xNorm2/1

== system StereoImageRectificationHDL/HDLStereoImageRectification/LeftUndistortion/RadialDistortion ==
  r4 : Inport
  r2 : Inport  Port=2
  Add3 : Sum
  Delay{10..13,18} (5 alike) : Delay
  Product1 : Product  OutDataTypeStr=Inherit: Same as first input
  Product2 : Product  OutDataTypeStr=Inherit: Same as first input
  radial1 : Constant  Value=distCoeffs(1)  OutDataTypeStr=fixdt(1,17,16)  SampleTime=-1
  radial2 : Constant  Value=distCoeffs(2)  OutDataTypeStr=fixdt(1,17,16)  SampleTime=-1
  alpha : Outport
  wires:
  r2/1 -> Delay10/1
  Add3/1 -> Delay18/1  "alpha"
  Product1/1 -> Delay13/1
  Delay13/1 -> Add3/2
  radial2/1 -> Product2/2
  r4/1 -> Delay11/1
  Product2/1 -> Delay12/1
  Delay11/1 -> Product2/1
  Delay18/1 -> alpha/1
  radial1/1 -> Product1/2
  Delay12/1 -> Add3/1
  Delay10/1 -> Product1/1

== system StereoImageRectificationHDL/HDLStereoImageRectification/LeftUndistortion/dxTangential ==
  r2 : Inport
  xyProd : Inport  Port=2
  xNorm2 : Inport  Port=3
  Add : Sum
  Add1 : Sum
  Delay{,1..4,6..7} (7 alike) : Delay
  Delay5 : Delay  DelayLength=1
  Product : Product  OutDataTypeStr=Inherit: Same as first input
  Product2 : Product  OutDataTypeStr=Inherit: Same as first input  LockScale=on
  Shift Arithmetic : ArithShift  BitShiftNumber=1  BitShiftDirection=Left
  Shift Arithmetic1 : ArithShift  BitShiftNumber=1  BitShiftDirection=Left
  tangential1 : Constant  Value=distCoeffs(3)  OutDataTypeStr=fixdt(1,17,15)  SampleTime=-1
  tangential2 : Constant  Value=distCoeffs(4)  OutDataTypeStr=fixdt(1,17,15)  SampleTime=-1
  dxTan : Outport
  wires:
  xyProd/1 -> Product/1
  xNorm2/1 -> Shift Arithmetic/1
  Shift Arithmetic/1 -> Delay/1
  Delay/1 -> Add/1
  r2/1 -> Delay1/1
  Delay1/1 -> Add/2
  Add/1 -> Delay2/1
  Delay2/1 -> Product2/1
  tangential2/1 -> Product2/2
  Product/1 -> Delay6/1
  Delay3/1 -> Add1/1
  Product2/1 -> Delay4/1
  Delay4/1 -> Add1/2
  Add1/1 -> Delay5/1
  Delay5/1 -> dxTan/1
  Shift Arithmetic1/1 -> Delay7/1
  tangential1/1 -> Product/2
  Delay6/1 -> Shift Arithmetic1/1
  Delay7/1 -> Delay3/1

== system StereoImageRectificationHDL/HDLStereoImageRectification/LeftUndistortion/dyTangential ==
  r2 : Inport
  xyProd : Inport  Port=2
  yNorm2 : Inport  Port=3
  Add : Sum
  Add1 : Sum
  Delay{,1..4,6..7} (7 alike) : Delay
  Delay5 : Delay  DelayLength=1
  Product : Product  OutDataTypeStr=Inherit: Same as first input
  Product2 : Product  OutDataTypeStr=Inherit: Same as first input
  Shift Arithmetic : ArithShift  BitShiftNumber=1  BitShiftDirection=Left
  Shift Arithmetic1 : ArithShift  BitShiftNumber=1  BitShiftDirection=Left
  tangential1 : Constant  Value=distCoeffs(3)  OutDataTypeStr=fixdt(1,17,15)  SampleTime=-1
  tangential2 : Constant  Value=distCoeffs(4)  OutDataTypeStr=fixdt(1,17,15)  SampleTime=-1
  dyTan : Outport
  wires:
  xyProd/1 -> Product/1
  tangential2/1 -> Product/2
  yNorm2/1 -> Shift Arithmetic/1
  Shift Arithmetic/1 -> Delay/1
  Delay/1 -> Add/1
  r2/1 -> Delay1/1
  Delay1/1 -> Add/2
  Add/1 -> Delay2/1
  Delay2/1 -> Product2/1
  tangential1/1 -> Product2/2
  Delay3/1 -> Add1/1
  Product2/1 -> Delay4/1
  Delay4/1 -> Add1/2
  Add1/1 -> Delay5/1
  Delay5/1 -> dyTan/1
  Shift Arithmetic1/1 -> Delay7/1
  Product/1 -> Delay6/1
  Delay6/1 -> Shift Arithmetic1/1
  Delay7/1 -> Delay3/1

== system StereoImageRectificationHDL/HDLStereoImageRectification/RightInterpolation/AddressGeneration ==
  u : Inport
  v : Inport  Port=2
  ctrl : Inport  Port=3
  Add : Sum  Inputs=+-  OutDataTypeStr=Inherit: Inherit via back propagation
  Add1 : Sum  Inputs=+-  OutDataTypeStr=Inherit: Inherit via back propagation
  AddressCalculation : Subsystem
  Data Type Conversion : DataTypeConversion  OutDataTypeStr=fixdt(0,max(ceil(log2(max(dimOut))),16),0)  SaturateOnIntegerOverflow=off  RndMeth=Floor
  Data Type Conversion1 : DataTypeConversion  OutDataTypeStr=fixdt(0,max(ceil(log2(max(dimOut))),16),0)  SaturateOnIntegerOverflow=off  RndMeth=Floor
  Delay{,1..3,7} (5 alike) : Delay  DelayLength=1
  Delay4 : Delay  DelayLength=4+1+3+3+10
  Delay5 : Delay  DelayLength=4+3+3+10
  Delay6 : Delay  DelayLength=4+3+3+10
  deltaU : Outport
  leftAdd : Outport  Port=2
  index : Outport  Port=3
  deltaV : Outport  Port=4
  ctrlOut : Outport  Port=5
  wires:
  v/1 -> Delay2/1, Data Type Conversion1/1
  Data Type Conversion1/1 -> Delay3/1, AddressCalculation/2(row)
  Data Type Conversion/1 -> Delay1/1, AddressCalculation/1(col)
  u/1 -> Delay/1, Data Type Conversion/1
  Delay/1 -> Add/1
  Delay1/1 -> Add/2
  Add/1 -> Delay6/1  "deltaU"
  Delay3/1 -> Add1/2
  Add1/1 -> Delay5/1  "deltaV"
  Delay2/1 -> Add1/1
  AddressCalculation/1(leftAdd) -> leftAdd/1
  AddressCalculation/2(leftIndex) -> Delay7/1
  ctrl/1 -> Delay4/1
  Delay6/1 -> deltaU/1
  Delay7/1 -> index/1
  Delay5/1 -> deltaV/1
  Delay4/1 -> ctrlOut/1

== system StereoImageRectificationHDL/HDLStereoImageRectification/RightInterpolation/BilinearInterpolation ==
  deltaU : Inport
  pixValue : Inport  Port=2
  Index : Inport  Port=3
  deltaV : Inport  Port=4
  ctrlIn : Inport  Port=5
  BilinearInterpolationEquation : Subsystem
  Constant : Constant  Value=0  OutDataTypeStr=Inherit: Inherit via back propagation  SampleTime=-1
  Delay8 : Delay  DelayLength=8
  IndexChangeForInterpolation : MATLAB Function  TreatAsAtomicUnit=on
  Pixel Control Bus Selector : BusSelector  OutputSignals=valid
  Switch : Switch  Criteria=u2 ~= 0  SaturateOnIntegerOverflow=off  InputSameDT=off
  rightPixel : Outport
  rightctrl : Outport  Port=2
  wires:
  Switch/1 -> rightPixel/1
  IndexChangeForInterpolation/1(pixOut) -> BilinearInterpolationEquation/2(pixValue)
  Constant/1 -> Switch/3
  pixValue/1 -> IndexChangeForInterpolation/1(pixelValue)
  BilinearInterpolationEquation/1(leftPixel) -> Switch/1
  Pixel Control Bus Selector/1 -> Switch/2  "<valid>"
  Delay8/1 -> rightctrl/1, Pixel Control Bus Selector/1
  deltaU/1 -> BilinearInterpolationEquation/1(deltaU)
  deltaV/1 -> BilinearInterpolationEquation/3(deltaV)
  Index/1 -> IndexChangeForInterpolation/2(index)
  ctrlIn/1 -> Delay8/1

== system StereoImageRectificationHDL/HDLStereoImageRectification/RightInterpolation/CacheMemory ==
  rightPixel1 : Inport
  rightCtrl1 : Inport  Port=2
  rightReadAddr : Inport  Port=3
  Data Type Conversion1 : DataTypeConversion  OutDataTypeStr=fixdt(0,ceil(log2(offset*dimOut(2)/4)),0)  SaturateOnIntegerOverflow=off  RndMeth=Floor
  RightWriteControl : Subsystem
  Simple Dual Port RAM System1 : hdlsllib/HDL RAMs/Simple Dual Port RAM System  RAMType=Simple dual port  WriteOutputValue=New data  RAMInitialValue=0  SimulateUsing=Code generation
      settings: SourceProductBaseCode=SL
  rightPixValue : Outport  VectorParamsAs1DForOutWhenUnconnected=off
  wires:
  rightReadAddr/1 -> Data Type Conversion1/1
  RightWriteControl/1(din) -> Simple Dual Port RAM System1/1  "din"
  rightPixel1/1 -> RightWriteControl/1(rightPixel)
  RightWriteControl/3(wr_en) -> Simple Dual Port RAM System1/3  "wrEN"
  Simple Dual Port RAM System1/1 -> rightPixValue/1  "pixValue"
  RightWriteControl/2(wr_addr) -> Simple Dual Port RAM System1/2  "WA"
  rightCtrl1/1 -> RightWriteControl/2(rightCtrl)
  Data Type Conversion1/1 -> Simple Dual Port RAM System1/4  "RA"

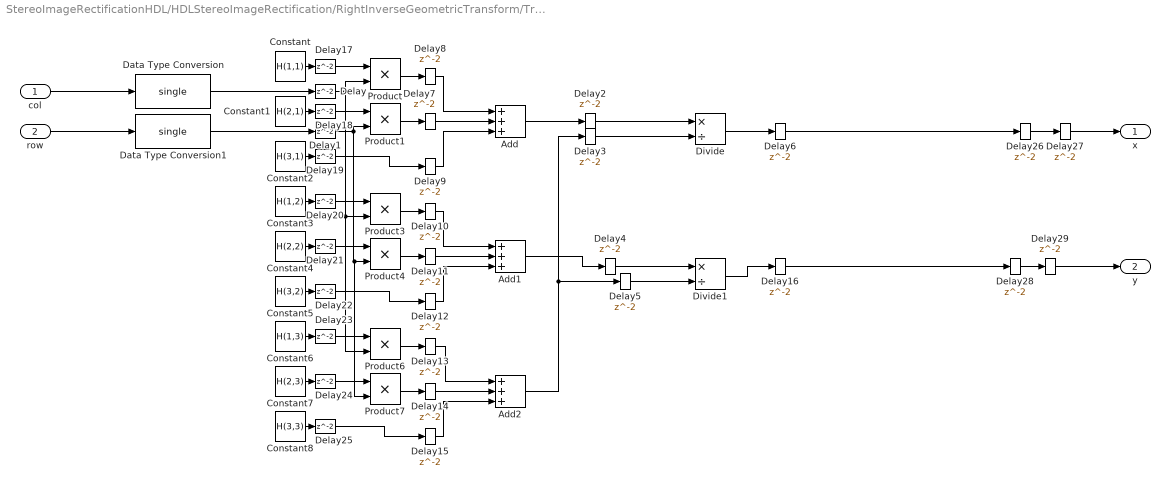
== system StereoImageRectificationHDL/HDLStereoImageRectification/RightInverseGeometricTransform/Transformation ==
  col : Inport
  row : Inport  Port=2
  Add : Sum  Inputs=3  RndMeth=Round
  Add1 : Sum  Inputs=3  RndMeth=Round
  Add2 : Sum  Inputs=3  RndMeth=Round
  Constant : Constant  Value=H(1,1)  OutDataTypeStr=single  SampleTime=-1
  Constant1 : Constant  Value=H(2,1)  OutDataTypeStr=single  SampleTime=-1
  Constant2 : Constant  Value=H(3,1)  OutDataTypeStr=single  SampleTime=-1
  Constant3 : Constant  Value=H(1,2)  OutDataTypeStr=single  SampleTime=-1
  Constant4 : Constant  Value=H(2,2)  OutDataTypeStr=single  SampleTime=-1
  Constant5 : Constant  Value=H(3,2)  OutDataTypeStr=single  SampleTime=-1
  Constant6 : Constant  Value=H(1,3)  OutDataTypeStr=single  SampleTime=-1
  Constant7 : Constant  Value=H(2,3)  OutDataTypeStr=single  SampleTime=-1
  Constant8 : Constant  Value=H(3,3)  OutDataTypeStr=single  SampleTime=-1
  Data Type Conversion : DataTypeConversion  OutDataTypeStr=single  SaturateOnIntegerOverflow=off  RndMeth=Floor
  Data Type Conversion1 : DataTypeConversion  OutDataTypeStr=single  SaturateOnIntegerOverflow=off  RndMeth=Floor
  Delay{,1..29} (30 alike) : Delay
  Divide : Product  Inputs=*/
  Divide1 : Product  Inputs=*/
  Product{,1,3..4,6..7} (6 alike) : Product  RndMeth=Round
  x : Outport
  y : Outport  Port=2
  wires:
  Constant5/1 -> Delay22/1
  Product/1 -> Delay8/1
  Delay12/1 -> Add1/3
  Constant1/1 -> Delay18/1
  Constant6/1 -> Delay23/1
  Add2/1 -> Delay3/1, Delay5/1
  Constant3/1 -> Delay20/1
  Delay13/1 -> Add2/1
  Constant4/1 -> Delay21/1
  Delay21/1 -> Product4/1
  Add/1 -> Delay2/1
  Delay10/1 -> Add1/1
  Delay9/1 -> Add/3
  Delay25/1 -> Delay15/1
  Delay1/1 -> Product7/2, Product4/2, Product1/2
  Delay7/1 -> Add/2
  Delay14/1 -> Add2/2
  Delay/1 -> Product/2, Product6/2, Product3/2
  Delay15/1 -> Add2/3
  Product6/1 -> Delay13/1
  Constant7/1 -> Delay24/1
  Delay11/1 -> Add1/2
  Delay22/1 -> Delay12/1
  Constant2/1 -> Delay19/1
  Product4/1 -> Delay11/1
  Constant/1 -> Delay17/1
  Product1/1 -> Delay7/1
  Delay17/1 -> Product/1
  Product3/1 -> Delay10/1
  Product7/1 -> Delay14/1
  Delay20/1 -> Product3/1
  Delay24/1 -> Product7/1
  Delay18/1 -> Product1/1
  col/1 -> Data Type Conversion/1
  Delay19/1 -> Delay9/1
  Delay8/1 -> Add/1
  Constant8/1 -> Delay25/1
  Delay23/1 -> Product6/1
  row/1 -> Data Type Conversion1/1
  Data Type Conversion/1 -> Delay/1
  Data Type Conversion1/1 -> Delay1/1
  Delay6/1 -> Delay26/1
  Delay16/1 -> Delay28/1
  Divide/1 -> Delay6/1
  Divide1/1 -> Delay16/1
  Add1/1 -> Delay4/1
  Delay2/1 -> Divide/1
  Delay3/1 -> Divide/2
  Delay4/1 -> Divide1/1
  Delay5/1 -> Divide1/2
  Delay26/1 -> Delay27/1
  Delay27/1 -> x/1
  Delay28/1 -> Delay29/1
  Delay29/1 -> y/1
